simulink model "playback_data"  (R2015a)
settings: Solver=FixedStepDiscrete  SolverMode=SingleTasking  StartTime=76  StopTime=110  FixedStep=sample_time  RelTol=1e-3
undefined symbols (not defined in the file): A1_notch_f1, A2_notch_f1, A_kalman_swing_load, A_kalman_transverse, A_kalman_vertical, A_lpf_accelerometer, A_lpf_dtau, A_lpf_fourbar_angles, A_lpf_imu, A_lpf_lateral_angle, B1_lpf_accelerometer, B1_lpf_dtau, B1_lpf_fourbar_angles, B1_lpf_imu, B1_lpf_lateral_angle, B1_notch_f1, B2_lpf_accelerometer, B2_lpf_dtau, B2_lpf_fourbar_angles, B2_lpf_imu, B2_lpf_lateral_angle, B2_notch_f1, B_dx_versus_x0, B_kalman_swing_load, B_kalman_transverse, B_kalman_vertical, backwards_K_sag_of_t, backwards_P_sag_of_t, C_kalman_swing_load, C_kalman_transverse, C_kalman_vertical, com_leg_motor, com_torso, contact_threshold, control_start_time, d_ankle_to_foot, d_vertical_com, desired_com_forward_velocity, desired_com_lateral_velocity, desired_initial_leg_roll_left, desired_initial_leg_roll_right, desired_stance_beta2, desired_standing_torso_pitch, desired_standing_torso_roll, desired_standing_z, desired_torso_pitch, desired_torso_roll, Discrete, enable_bouncing, fcut_contact, fdesignblkfcn, forward_dx_of_dxstar, forward_x_of_dxstar, g, gcbh, HIP_MTR_MAX_CONT_TORQUE, HIP_MTR_MAX_TORQUE, i_leg_motor, i_robot, i_torso ... (+78)
libraries: simulink x65, dsparch4 x18, ctrlSharedLib x14, dspfdesign x4
(part 7 of 13)

== system playback_data/Control/Actuator Control with Torque SEA commands/SEA Controller (Velocity)/Lowpass Filter (Stance) ==
  In : Inport
  Generated Filter Block : DiscreteFir  Tag=BlockMethodSubSystem  Coefficients=[-0.049792265798371309 -0.00478204397482343 -0.0023545966524627579 0.0019617877955006649 0.0081617445920188422 0.01606136498204886 0.025426522925330174 0.035808512742994333 0.046780148761454213 0.057713212050140641 0.068077289761393753 0.077169075575072327 0.084565882051693325 0.089692876147162801 0.092473878579640248 0.092473878579640248 0.089692876147162801 0.084565882051693325 0.077169075575072327 0.068077289761393753 0.057713212050140641 0.046780148761454213 0.035808512742994333 0.025426522925330174 0.01606136498204886 0.0081617445920188422 0.0019617877955006649 -0.0023545966524627579 -0.00478204397482343 -0.049792265798371309]
  Out : Outport
  wires:
  In/1 -> Generated Filter Block/1
  Generated Filter Block/1 -> Out/1

== system playback_data/Control/Actuator Control with Torque SEA commands/SEA Controller (Velocity)/Lowpass Filter (Swing) ==
  In : Inport
  Generated Filter Block : dsparch4/Biquad Filter  Tag=BlockMethodSubSystem  IIRFiltStruct=Direct form II  CoeffSource=Specify via dialog  BiQuadCoeffs=[1.0218648663828083 -2 1.0218648663828083 1 -1.9114378222117407 0.91557643487411833]  a0Flag=Warning  IC=0  ICnum=0  ICden=0  denAccumFracLength=30  denProdOutputFracLength=30  secondMemoryFracLength=15  roundingMode=Floor  overflowMode=off  ScaleValues=[0.0041174265739107223;22.985401576126357]  optimizeScaleValues=off  ScaleValueMode=Specify via input port (g)  scaleValueFracLength=14  FilterSource=Specify via dialog  FilterObject=Hm_biquad
  Out : Outport
  wires:
  Generated Filter Block/1 -> Out/1
  In/1 -> Generated Filter Block/1

== system playback_data/Control/Actuator Control with Torque SEA commands/SEA Controller (Velocity)/Stance or Swing ==
  True/False x4 : Inport
  Signal True x4 : Inport  Port=2
  Signal False x4 : Inport  Port=3
  Demux : Demux
  Demux1 : Demux
  Demux2 : Demux
  Mux : Mux
  Switch{,1..3} (4 alike) : Switch  Criteria=u2 ~= 0
  Selected x4 : Outport
  wires:
  Mux/1 -> Selected x4/1
  True/False x4/1 -> Demux1/1
  Signal True x4/1 -> Demux/1
  Signal False x4/1 -> Demux2/1
  Demux/1 -> Switch/1
  Demux/2 -> Switch1/1
  Demux/3 -> Switch2/1
  Demux/4 -> Switch3/1
  Demux2/1 -> Switch/3
  Demux2/2 -> Switch1/3
  Demux2/3 -> Switch2/3
  Demux2/4 -> Switch3/3
  Demux1/1 -> Switch/2
  Demux1/2 -> Switch1/2
  Demux1/3 -> Switch2/2
  Demux1/4 -> Switch3/2
  Switch/1 -> Mux/1
  Switch1/1 -> Mux/2
  Switch2/1 -> Mux/3
  Switch3/1 -> Mux/4

== system playback_data/Control/Actuator Control with Torque SEA commands/SEA Controller (Velocity)/Stance or Swing1 ==
  True/False x4 : Inport
  Signal True x4 : Inport  Port=2
  Signal False x4 : Inport  Port=3
  Demux : Demux
  Demux1 : Demux
  Demux2 : Demux
  Mux : Mux
  Switch{,1..3} (4 alike) : Switch  Criteria=u2 ~= 0
  Selected x4 : Outport
  wires:
  Switch3/1 -> Mux/4
  Switch2/1 -> Mux/3
  Switch1/1 -> Mux/2
  Switch/1 -> Mux/1
  Demux1/4 -> Switch3/2
  Demux1/3 -> Switch2/2
  Demux1/2 -> Switch1/2
  Demux1/1 -> Switch/2
  Demux2/4 -> Switch3/3
  Demux2/3 -> Switch2/3
  Demux2/2 -> Switch1/3
  Demux2/1 -> Switch/3
  Demux/4 -> Switch3/1
  Demux/3 -> Switch2/1
  Demux/2 -> Switch1/1
  Demux/1 -> Switch/1
  Signal False x4/1 -> Demux2/1
  Signal True x4/1 -> Demux/1
  True/False x4/1 -> Demux1/1
  Mux/1 -> Selected x4/1

== system playback_data/Control/Actuator Control with Torque SEA commands/SEA Controller (Velocity)/Stance or Swing2 ==
  True/False x4 : Inport
  Signal True x4 : Inport  Port=2
  Signal False x4 : Inport  Port=3
  Demux : Demux
  Demux1 : Demux
  Demux2 : Demux
  Mux : Mux
  Switch{,1..3} (4 alike) : Switch  Criteria=u2 ~= 0
  Selected x4 : Outport
  wires:
  Mux/1 -> Selected x4/1
  True/False x4/1 -> Demux1/1
  Signal True x4/1 -> Demux/1
  Signal False x4/1 -> Demux2/1
  Demux/1 -> Switch/1
  Demux/2 -> Switch1/1
  Demux/3 -> Switch2/1
  Demux/4 -> Switch3/1
  Demux2/1 -> Switch/3
  Demux2/2 -> Switch1/3
  Demux2/3 -> Switch2/3
  Demux2/4 -> Switch3/3
  Demux1/1 -> Switch/2
  Demux1/2 -> Switch1/2
  Demux1/3 -> Switch2/2
  Demux1/4 -> Switch3/2
  Switch/1 -> Mux/1
  Switch1/1 -> Mux/2
  Switch2/1 -> Mux/3
  Switch3/1 -> Mux/4

== system playback_data/Control/Actuator Control with Torque SEA commands/Timers/Time on Contact ==
  in : Inport
  Trigger : TriggerPort  ShowOutputPort=on  PortDimensions=1
  Subsystem : Subsystem
  out : Outport
  wires:
  in/1 -> Subsystem/1(in)
  Subsystem/1(out) -> out/1
  Trigger/1 -> Subsystem/Enable

== system playback_data/Control/Actuator Control with Torque SEA commands/Timers/Time on Contact1 ==
  in : Inport
  Trigger : TriggerPort  ShowOutputPort=on  PortDimensions=1
  Subsystem : Subsystem
  out : Outport
  wires:
  Trigger/1 -> Subsystem/Enable
  Subsystem/1(out) -> out/1
  in/1 -> Subsystem/1(in)

== system playback_data/Control/Actuator Control with Torque SEA commands/Timers/Time on Contact2 ==
  in : Inport
  Trigger : TriggerPort  ShowOutputPort=on  PortDimensions=1
  Subsystem : Subsystem
  out : Outport
  wires:
  Trigger/1 -> Subsystem/Enable
  Subsystem/1(out) -> out/1
  in/1 -> Subsystem/1(in)

== system playback_data/Control/Actuator Control with Torque SEA commands/Timers/Time on Contact3 ==
  in : Inport
  Trigger : TriggerPort  ShowOutputPort=on  PortDimensions=1
  Subsystem : Subsystem
  out : Outport
  wires:
  in/1 -> Subsystem/1(in)
  Subsystem/1(out) -> out/1
  Trigger/1 -> Subsystem/Enable

== system playback_data/Control/Behavior Control/Force Estimation/Leg Force Measurements ==
  q : Inport
  Leg Width Right/Left [m m] : Inport  Port=2
  Leg Length Right/Left [m m] : Inport  Port=3
  Demux : Demux  Outputs=2
  Demux1 : Demux  Outputs=2
  Demux2 : Demux
  Divide{1..4} (4 alike) : Product  Inputs=*/
  Gain : Gain  Commented=on  Gain=k_sea_low
  Mux : Mux
  Nonlinear Spring Force : MATLAB Function  TreatAsAtomicUnit=on
  Sum{1..3,6} (4 alike) : Sum  Inputs=-+|
  Sum4 : Sum  Inputs=-|+
  Sum5 : Sum  Inputs=-|+
  Sum7 : Sum  Inputs=+|+
  Sum8 : Sum  Inputs=+|+
  backGearL : Selector  InputPortWidth=13  Indices=[6]
  backGearR : Selector  InputPortWidth=13  Indices=[2]
  backJointL : Selector  InputPortWidth=13  Indices=[5]
  backJointR : Selector  InputPortWidth=13  Indices=[1]
  frontGearL : Selector  InputPortWidth=13  Indices=[8]
  frontGearR : Selector  InputPortWidth=13  Indices=[4]
  frontJointL : Selector  InputPortWidth=13  Indices=[7]
  frontJointR : Selector  InputPortWidth=13  Indices=[3]
  Right Leg Torque [Nm] : Outport
  Left Leg Torque [Nm] : Outport  Port=2
  Right Leg Axial Force [N] : Outport  Port=3
  Left Leg Axial Force [N] : Outport  Port=4
  Right Leg Orthogonal Force [N] : Outport  Port=5
  Left Leg Orthogonal Force [N] : Outport  Port=6
  wires:
  Sum3/1 -> Mux/4
  Sum2/1 -> Mux/3
  backJointL/1 -> Sum2/1
  frontGearL/1 -> Sum3/2
  frontJointL/1 -> Sum3/1
  backGearL/1 -> Sum2/2
  Sum6/1 -> Mux/1
  Sum1/1 -> Mux/2
  backJointR/1 -> Sum6/1
  frontGearR/1 -> Sum1/2
  frontJointR/1 -> Sum1/1
  backGearR/1 -> Sum6/2
  q/1 -> backGearR/1, backJointL/1, frontJointL/1, frontGearL/1, backGearL/1, frontGearR/1, frontJointR/1, backJointR/1
  Demux2/1 -> Sum4/1, Sum7/1
  Demux2/2 -> Sum7/2, Sum4/2
  Demux2/4 -> Sum5/2, Sum8/2
  Sum4/1 -> Divide1/1
  Sum5/1 -> Divide2/1
  Leg Width Right/Left [m m]/1 -> Demux/1
  Demux/1 -> Divide1/2
  Demux/2 -> Divide2/2
  Divide1/1 -> Right Leg Axial Force [N]/1
  Divide2/1 -> Left Leg Axial Force [N]/1
  Demux2/3 -> Sum8/1, Sum5/1
  Sum7/1 -> Divide3/1, Right Leg Torque [Nm]/1
  Sum8/1 -> Divide4/1, Left Leg Torque [Nm]/1
  Demux1/1 -> Divide3/2
  Demux1/2 -> Divide4/2
  Leg Length Right/Left [m m]/1 -> Demux1/1
  Divide3/1 -> Right Leg Orthogonal Force [N]/1
  Divide4/1 -> Left Leg Orthogonal Force [N]/1
  Mux/1 -> Nonlinear Spring Force/1(deflections)
  Nonlinear Spring Force/1(tau_sea) -> Demux2/1

== system playback_data/Control/Behavior Control/Force Estimation/Leg Plane GRF ==
  Axial Force [N] : Inport
  Orthogonal Force [N] : Inport  Port=2
  Torso Pitch [rad] : Inport  Port=3
  Leg Angle [rad] : Inport  Port=4
  Gain : Gain  Gain=-1
  Product : Product
  Product1 : Product
  Sum : Sum  Inputs=++|
  Sum1 : Sum  Inputs=+|+
  Trigonometric Function : Trigonometry  Operator=cos
  Trigonometric Function1 : Trigonometry
  Vertical Force [N] : Outport
  wires:
  Product1/1 -> Sum1/2
  Sum1/1 -> Vertical Force [N]/1
  Trigonometric Function1/1 -> Product1/2
  Orthogonal Force [N]/1 -> Product1/1
  Axial Force [N]/1 -> Product/1
  Leg Angle [rad]/1 -> Sum/2
  Torso Pitch [rad]/1 -> Sum/1
  Trigonometric Function/1 -> Product/2
  Product/1 -> Gain/1
  Sum/1 -> Trigonometric Function/1, Trigonometric Function1/1
  Gain/1 -> Sum1/1

== system playback_data/Control/Behavior Control/Primary and Lateral Behavior/Circular Buffer ==
  Flight [1/0] : Inport
  Exiting Stance [1/0] : Inport  Port=2
  Hopping [1/0] : Inport  Port=3
  dX [m/s] : Inport  Port=4
  dY [m/s] : Inport  Port=5
  X Foot Correction [m] : Inport  Port=6
  Y Foot Correction [m] : Inport  Port=7
  target dX [m/s] : Inport  Port=8
  target dY [m/s] : Inport  Port=9
  Buffer : MATLAB Function  TreatAsAtomicUnit=on  SystemSampleTime=sample_time
  Buffer1 : MATLAB Function  TreatAsAtomicUnit=on  SystemSampleTime=sample_time
  Buffer2 : MATLAB Function  TreatAsAtomicUnit=on  SystemSampleTime=sample_time
  Buffer3 : MATLAB Function  TreatAsAtomicUnit=on  SystemSampleTime=sample_time
  Buffer4 : MATLAB Function  TreatAsAtomicUnit=on  SystemSampleTime=sample_time
  Buffer5 : MATLAB Function  TreatAsAtomicUnit=on  SystemSampleTime=sample_time
  Buffer6 : MATLAB Function  TreatAsAtomicUnit=on  SystemSampleTime=sample_time
  Buffer7 : MATLAB Function  TreatAsAtomicUnit=on  SystemSampleTime=sample_time
  Demux : Demux  Outputs=6
  Detect Decrease : simulink/Logic and Bit Operations/Detect Decrease  vinit=0.0  InputProcessing=Inherited  OutDataTypeStr=boolean
  Enabled on Touchdown : Subsystem  TreatAsAtomicUnit=on
  Logical Operator : Logic  AllPortsSameDT=off  OutDataTypeStr=boolean
  Mux : Mux  Inputs=6
  buffer size5 : Constant  Value=recorded_steps
  "dX Touchdown History " : Outport
  X Foot Correction History : Outport  Port=2
  dX Takeoff History : Outport  Port=3
  "dY Touchdown History " : Outport  Port=4
  Y Foot Correction History : Outport  Port=5
  dY Takeoff History : Outport  Port=6
  target dX History : Outport  Port=7
  target dY History : Outport  Port=8
  wires:
  Enabled on Touchdown/1(Out) -> Demux/1
  Mux/1 -> Enabled on Touchdown/1(In)
  Logical Operator/1 -> Detect Decrease/1
  Flight [1/0]/1 -> Logical Operator/2
  dX [m/s]/1 -> Mux/1, Buffer2/1(data)
  dY [m/s]/1 -> Mux/2, Buffer5/1(data)
  Hopping [1/0]/1 -> Logical Operator/1
  Exiting Stance [1/0]/1 -> Buffer5/2(trigger), Buffer2/2(trigger), Buffer3/2(trigger), Buffer1/2(trigger), Buffer4/2(trigger), Buffer6/2(trigger), Buffer7/2(trigger), Buffer/2(trigger)
  target dY [m/s]/1 -> Mux/6
  Demux/5 -> Buffer6/1(data)
  Demux/6 -> Buffer7/1(data)
  buffer size5/1 -> Buffer5/3(buffer_size), Buffer3/3(buffer_size), Buffer1/3(buffer_size), Buffer4/3(buffer_size), Buffer6/3(buffer_size), Buffer7/3(buffer_size), Buffer/3(buffer_size), Buffer2/3(buffer_size)
  Buffer7/1(buffer) -> target dY History/1
  Buffer6/1(buffer) -> target dX History/1
  target dX [m/s]/1 -> Mux/5
  Demux/4 -> Buffer4/1(data)
  Y Foot Correction [m]/1 -> Mux/4
  Buffer5/1(buffer) -> dY Takeoff History/1
  Demux/2 -> Buffer3/1(data)
  Buffer4/1(buffer) -> Y Foot Correction History/1
  Buffer3/1(buffer) -> "dY Touchdown History "/1
  X Foot Correction [m]/1 -> Mux/3
  Demux/3 -> Buffer1/1(data)
  Demux/1 -> Buffer/1(data)
  Buffer2/1(buffer) -> dX Takeoff History/1
  Buffer1/1(buffer) -> X Foot Correction History/1
  Detect Decrease/1 -> Enabled on Touchdown/Enable
  Buffer/1(buffer) -> "dX Touchdown History "/1

== system playback_data/Control/Behavior Control/Primary and Lateral Behavior/Closed Loop Compensation ==
  dX Touchdown History : Inport
  X Foot Correction History : Inport  Port=2
  dX Takeoff History : Inport  Port=3
  dY Touchdown History : Inport  Port=4
  Y Foot Correction History : Inport  Port=5
  dY Takeoff History : Inport  Port=6
  target dX History : Inport  Port=7
  target dY History : Inport  Port=8
  dX [m/s] : Inport  Port=9
  dY [m/s] : Inport  Port=10
  target dX [m/s] : Inport  Port=11
  "target dY [m/s] " : Inport  Port=12
  A_x : Gain
  A_x_no_bias : Gain
  A_y : Gain
  A_y_no_bias : Gain
  CLOSED LOOP COMPENSATION X FOR VAIRABLE SPEED : MATLAB Function  TreatAsAtomicUnit=on
  CLOSED LOOP COMPENSATION Y FOR VAIRABLE SPEED : MATLAB Function  TreatAsAtomicUnit=on
  Constant4 : Constant  Value=B_dx_versus_x0
  ESTIMATE CLOSED LOOP ERROR X FOR VARIABLE SPEED : MATLAB Function  TreatAsAtomicUnit=on
  ESTIMATE CLOSED LOOP ERROR Y FOR VARIABLE SPEED : MATLAB Function  TreatAsAtomicUnit=on
  How much dx depends on x0 : Constant  Value=B_dx_versus_x0
  RealVsFakeWeight : Constant  Value=2
  RealVsFakeWeight1 : Constant  Value=2
  Sum : Sum  Inputs=|+-
  Sum1 : Sum  Inputs=|+-
  Terminator{2..12,14} (12 alike) : Terminator
  XY Foot Correction : Scope  NumInputPorts=2
      settings: YMin=-1~-0.8  YMax=1~1.4  SaveName=ScopeData39  SampleInput=on
  c_x : Gain
  c_x_no_bias : Gain
  c_y : Gain
  c_y_no_bias : Gain
  epsilon_x : Gain
  epsilon_x_no_bias : Gain
  epsilon_y : Gain
  epsilon_y_no_bias : Gain
  X Foot Correction [m] : Outport
  Y Foot Correction [m] : Outport  Port=2
  wires:
  RealVsFakeWeight1/1 -> ESTIMATE CLOSED LOOP ERROR Y FOR VARIABLE SPEED/5(W_real)
  Constant4/1 -> CLOSED LOOP COMPENSATION Y FOR VAIRABLE SPEED/6(B_cl)
  "target dY [m/s] "/1 -> Sum1/2, CLOSED LOOP COMPENSATION Y FOR VAIRABLE SPEED/5(dx_star)
  target dY History/1 -> ESTIMATE CLOSED LOOP ERROR Y FOR VARIABLE SPEED/4(dx_star_hist)
  Y Foot Correction History/1 -> ESTIMATE CLOSED LOOP ERROR Y FOR VARIABLE SPEED/2(delta_ux_hist)
  dY Takeoff History/1 -> ESTIMATE CLOSED LOOP ERROR Y FOR VARIABLE SPEED/3(dx_lift_hist)
  dY [m/s]/1 -> Sum1/1
  RealVsFakeWeight/1 -> ESTIMATE CLOSED LOOP ERROR X FOR VARIABLE SPEED/5(W_real)
  How much dx depends on x0/1 -> CLOSED LOOP COMPENSATION X FOR VAIRABLE SPEED/6(B_cl)
  Sum/1 -> CLOSED LOOP COMPENSATION X FOR VAIRABLE SPEED/4(delta_s_i)
  target dX [m/s]/1 -> Sum/2, CLOSED LOOP COMPENSATION X FOR VAIRABLE SPEED/5(dx_star)
  target dX History/1 -> ESTIMATE CLOSED LOOP ERROR X FOR VARIABLE SPEED/4(dx_star_hist)
  X Foot Correction History/1 -> ESTIMATE CLOSED LOOP ERROR X FOR VARIABLE SPEED/2(delta_ux_hist)
  dX Takeoff History/1 -> ESTIMATE CLOSED LOOP ERROR X FOR VARIABLE SPEED/3(dx_lift_hist)
  dX Touchdown History/1 -> ESTIMATE CLOSED LOOP ERROR X FOR VARIABLE SPEED/1(dx_land_hist)
  dX [m/s]/1 -> Sum/1
  dY Touchdown History/1 -> ESTIMATE CLOSED LOOP ERROR Y FOR VARIABLE SPEED/1(dx_land_hist)
  Sum1/1 -> CLOSED LOOP COMPENSATION Y FOR VAIRABLE SPEED/4(delta_s_i)
  CLOSED LOOP COMPENSATION X FOR VAIRABLE SPEED/1(delta_ux) -> XY Foot Correction/1, X Foot Correction [m]/1
  CLOSED LOOP COMPENSATION Y FOR VAIRABLE SPEED/1(delta_ux) -> XY Foot Correction/2, Y Foot Correction [m]/1
  ESTIMATE CLOSED LOOP ERROR X FOR VARIABLE SPEED/6(c_nb) -> c_x_no_bias/1
  ESTIMATE CLOSED LOOP ERROR X FOR VARIABLE SPEED/5(epsilon_0_nb) -> epsilon_x_no_bias/1
  ESTIMATE CLOSED LOOP ERROR X FOR VARIABLE SPEED/4(A_cl_nb) -> A_x_no_bias/1
  A_x_no_bias/1 -> Terminator5/1
  epsilon_x_no_bias/1 -> Terminator6/1
  c_x_no_bias/1 -> Terminator7/1
  A_y_no_bias/1 -> Terminator2/1
  epsilon_y_no_bias/1 -> Terminator3/1
  c_y_no_bias/1 -> Terminator4/1
  ESTIMATE CLOSED LOOP ERROR Y FOR VARIABLE SPEED/4(A_cl_nb) -> A_y_no_bias/1
  ESTIMATE CLOSED LOOP ERROR Y FOR VARIABLE SPEED/5(epsilon_0_nb) -> epsilon_y_no_bias/1
  ESTIMATE CLOSED LOOP ERROR Y FOR VARIABLE SPEED/6(c_nb) -> c_y_no_bias/1
  ESTIMATE CLOSED LOOP ERROR X FOR VARIABLE SPEED/3(c) -> c_x/1, CLOSED LOOP COMPENSATION X FOR VAIRABLE SPEED/3(c)
  ESTIMATE CLOSED LOOP ERROR X FOR VARIABLE SPEED/2(epsilon_0) -> epsilon_x/1, CLOSED LOOP COMPENSATION X FOR VAIRABLE SPEED/2(epsilon)
  ESTIMATE CLOSED LOOP ERROR X FOR VARIABLE SPEED/1(A_cl) -> A_x/1, CLOSED LOOP COMPENSATION X FOR VAIRABLE SPEED/1(A_cl)
  A_x/1 -> Terminator8/1
  epsilon_x/1 -> Terminator9/1
  c_x/1 -> Terminator10/1
  ESTIMATE CLOSED LOOP ERROR Y FOR VARIABLE SPEED/3(c) -> c_y/1, CLOSED LOOP COMPENSATION Y FOR VAIRABLE SPEED/3(c)
  ESTIMATE CLOSED LOOP ERROR Y FOR VARIABLE SPEED/2(epsilon_0) -> epsilon_y/1, CLOSED LOOP COMPENSATION Y FOR VAIRABLE SPEED/2(epsilon)
  ESTIMATE CLOSED LOOP ERROR Y FOR VARIABLE SPEED/1(A_cl) -> A_y/1, CLOSED LOOP COMPENSATION Y FOR VAIRABLE SPEED/1(A_cl)
  A_y/1 -> Terminator12/1
  epsilon_y/1 -> Terminator14/1
  c_y/1 -> Terminator11/1

== system playback_data/Control/Behavior Control/Primary and Lateral Behavior/Enabled on Takeoff ==
  In : Inport
  Enable : EnablePort
  Out : Outport
  wires:
  In/1 -> Out/1

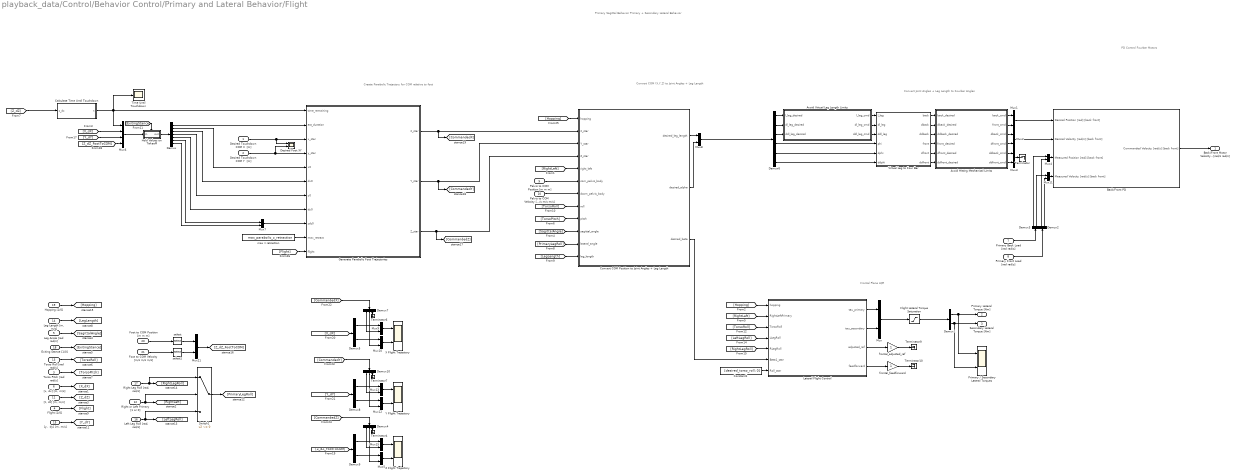
== system playback_data/Control/Behavior Control/Primary and Lateral Behavior/Flight ==
  note: Primary Sagittal Behavior
      | Primary + Secondary Lateral Behavior
  note: Create Parabolic
      | Trajectory for COM relative to foot
  note: Convert COM (X,Y,Z) to
      | Joint Angles + Leg Length
  note: Convert Joint Angles + Leg Length
      | to Fourbar Angles
  note: PD Control Fourbar Motors
  note: Frontal Plane LQR
  Desired Touchdown COM X  [m] : Inport
  Desired Touchdown COM Y  [m] : Inport  Port=2
  Torso Pitch [rad rad/s] : Inport  Port=3
  Flight [1/0] : Inport  Port=4
  Leg Angle [rad rad/s] : Inport  Port=5
  "[x, dx] [m, m/s]" : Inport  Port=6
  Primary Back Load [rad rad/s] : Inport  Port=7
  Primary Front Load [rad rad/s] : Inport  Port=8
  Pelvis to COM Position [m m m] : Inport  Port=9
  Pelvis to COM Velocity [m/s m/s m/s] : Inport  Port=10
  "[z, dz] [m, m/s]" : Inport  Port=11
  Right or Left Primary [1 or 0] : Inport  Port=12
  Torso Roll [rad rad/s] : Inport  Port=13
  "Leg Length [m, m/s]" : Inport  Port=14
  "[y,  dy] [m, m/s]" : Inport  Port=15
  "Left Leg Roll [rad, rad/s]" : Inport  Port=16
  "Right Leg Roll [rad, rad/s]" : Inport  Port=17
  Exiting Stance [1/0] : Inport  Port=18
  Hopping [1/0] : Inport  Port=19
  Foot to COM Position [m m m] : Inport  Port=20
  Foot to COM Velocity [m/s m/s m/s] : Inport  Port=21
  Avoid Hitting Mechanical Limits : MATLAB Function  TreatAsAtomicUnit=on
  Avoid Virtual Leg Length Limits : MATLAB Function  TreatAsAtomicUnit=on
  Back/Front PD : Subsystem
  Calculate Time Until Touchdown : MATLAB Function  TreatAsAtomicUnit=on
  Constant1 : Constant  Value=[desired_torso_roll; 0]
  "Convert COM Position to Joint Angles + Leg Length " : MATLAB Function  TreatAsAtomicUnit=on
  Demux : Demux  Outputs=7
  Demux{1..3,5,8..9} (6 alike) : Demux  Outputs=2
  Demux10 : Demux  Outputs=3
  Demux4 : Demux  Outputs=3
  Demux6 : Demux  Outputs=6
  Demux7 : Demux  Outputs=3
  Desired Foot XY : Scope  NumInputPorts=2
      settings: YMin=-1~-0.8  YMax=1~1.4  SaveName=ScopeData38  SampleInput=on
  Flight Lateral Torque Saturation : Saturate  UpperLimit=HIP_MTR_MAX_CONT_TORQUE  LowerLimit=-HIP_MTR_MAX_CONT_TORQUE
      settings: AttributesFormatString=Top: %<UpperLimit>\nBottom: %<LowerLimit>
  Generate Parabolic Foot Trajectories : MATLAB Function  TreatAsAtomicUnit=on
  Hold Values on Takeoff : Subsystem
  Lateral Flight Control : MATLAB Function  TreatAsAtomicUnit=on
  Mux{,1..5,7..13,15,21} (15 alike) : Mux  Inputs=2
  Mux6 : Mux
  Primary / Secondary Lateral Torques : Scope  NumInputPorts=2
      settings: YMin=-1~-0.8  YMax=1~1.4  SaveName=ScopeData32  SampleInput=on
  Switch1 : Switch  Criteria=u2 ~= 0
  Terminator{,4,6..7,9..10} (6 alike) : Terminator
  Time Until Touchdown : Scope
      settings: YMin=-1  YMax=1  SaveName=ScopeData37  SampleInput=on
  Virtual Leg to Four Bar : MATLAB Function  TreatAsAtomicUnit=on
  X Flight Trajectory : Scope  NumInputPorts=2
      settings: YMin=-1~-0.8  YMax=1~1.4  SaveName=ScopeData3  SampleInput=on
  Y Flight Trajectory : Scope  NumInputPorts=2
      settings: YMin=-1~-0.8  YMax=1~1.4  SaveName=ScopeData4  SampleInput=on
  Z Flight Trajectory : Scope  NumInputPorts=2
      settings: YMin=-1~-0.8  YMax=1~1.4  SaveName=ScopeData7  SampleInput=on
  frontal_adjusted_ref : Gain
  frontal_feedforward : Gain
  max z retraction : Constant  Value=max_parabolic_z_retraction
  select : Selector  InputPortWidth=3  Indices=[3]
  select1 : Selector  InputPortWidth=3  Indices=[3]
  Back/Front Motor Velocity [rad/s rad/s] : Outport
  Primary Lateral Torque [Nm] : Outport  Port=2
  Secondary Lateral Torque [Nm] : Outport  Port=3
  wires:
  Virtual Leg to Four Bar/1(back) -> Avoid Hitting Mechanical Limits/1(back_desired)
  Virtual Leg to Four Bar/2(dback) -> Avoid Hitting Mechanical Limits/2(dback_desired)
  Virtual Leg to Four Bar/3(ddback) -> Avoid Hitting Mechanical Limits/3(ddback_desired)
  Virtual Leg to Four Bar/4(front) -> Avoid Hitting Mechanical Limits/4(front_desired)
  Virtual Leg to Four Bar/5(dfront) -> Avoid Hitting Mechanical Limits/5(dfront_desired)
  Virtual Leg to Four Bar/6(ddfront) -> Avoid Hitting Mechanical Limits/6(ddfront_desired)
  Mux11/1 -> Back/Front PD/4(Measured Velocity [rad/s] [back front])
  Demux2/2 -> Mux11/2
  Mux4/1 -> Back/Front PD/3(Measured Position [rad] [back front])
  Mux1/1 -> Back/Front PD/1(Desired Position [rad] [back front])
  Demux3/2 -> Mux11/1
  Demux3/1 -> Mux4/1
  Avoid Hitting Mechanical Limits/2(front_cmd) -> Mux1/2
  Avoid Hitting Mechanical Limits/1(back_cmd) -> Mux1/1
  Demux2/1 -> Mux4/2
  Avoid Hitting Mechanical Limits/3(dback_cmd) -> Mux2/1
  Avoid Hitting Mechanical Limits/4(dfront_cmd) -> Mux2/2
  Avoid Hitting Mechanical Limits/5(ddback_cmd) -> Mux3/1
  Avoid Hitting Mechanical Limits/6(ddfront_cmd) -> Mux3/2
  Mux2/1 -> Back/Front PD/2(Desired Velocity [rad/s] [back front])
  Back/Front PD/1(Commanded Velocity [rad/s] [back front]) -> Back/Front Motor Velocity [rad/s rad/s]/1
  Primary Back Load [rad rad/s]/1 -> Demux3/1
  Primary Front Load [rad rad/s]/1 -> Demux2/1
  Demux/1 -> Generate Parabolic Foot Trajectories/2(est_duration)
  Mux7/1 -> Generate Parabolic Foot Trajectories/9(zdz0)
  max z retraction/1 -> Generate Parabolic Foot Trajectories/10(max_retract)
  Mux6/1 -> Hold Values on Takeoff/1(in)
  Hold Values on Takeoff/1(out) -> Demux/1
  [X_dX] -> Mux6/2
  Generate Parabolic Foot Trajectories/1(X_star) -> [CommandedX], "Convert COM Position to Joint Angles + Leg Length "/2(X_star)
  Generate Parabolic Foot Trajectories/2(Y_star) -> "Convert COM Position to Joint Angles + Leg Length "/3(Y_star), [CommandedY]
  [RightLeft] -> "Convert COM Position to Joint Angles + Leg Length "/5(right_left)
  "Convert COM Position to Joint Angles + Leg Length "/2(desired_alpha) -> Mux8/2
  "Convert COM Position to Joint Angles + Leg Length "/1(desired_leg_length) -> Mux8/1
  Demux6/6 -> Virtual Leg to Four Bar/6(ddphi)
  Demux6/5 -> Virtual Leg to Four Bar/5(dphi)
  Demux6/4 -> Virtual Leg to Four Bar/4(phi)
  Mux8/1 -> Demux6/1
  Leg Angle [rad rad/s]/1 -> [SagittalAngle]
  [SagittalAngle] -> "Convert COM Position to Joint Angles + Leg Length "/10(sagittal_angle)
  Torso Pitch [rad rad/s]/1 -> [TorsoPitch]
  [TorsoPitch] -> "Convert COM Position to Joint Angles + Leg Length "/9(pitch)
  [PrimaryLegRoll] -> "Convert COM Position to Joint Angles + Leg Length "/11(lateral_angle)
  [LegLength] -> "Convert COM Position to Joint Angles + Leg Length "/12(leg_length)
  [TorsoRoll] -> "Convert COM Position to Joint Angles + Leg Length "/8(roll)
  Pelvis to COM Position [m m m]/1 -> "Convert COM Position to Joint Angles + Leg Length "/6(com_pelvis_body)
  Pelvis to COM Velocity [m/s m/s m/s]/1 -> "Convert COM Position to Joint Angles + Leg Length "/7(dcom_pelvis_body)
  Flight [1/0]/1 -> [Flight]
  [ExitingStance] -> Hold Values on Takeoff/Trigger
  "[x, dx] [m, m/s]"/1 -> [X_dX]
  Torso Roll [rad rad/s]/1 -> [TorsoRoll]
  "Leg Length [m, m/s]"/1 -> [LegLength]
  "[z, dz] [m, m/s]"/1 -> [Z_dZ]
  Desired Touchdown COM X  [m]/1 -> Desired Foot XY/1, Generate Parabolic Foot Trajectories/3(x_star)
  "[y,  dy] [m, m/s]"/1 -> [Y_dY]
  [Y_dY] -> Mux6/3
  [Z_dZ] -> Calculate Time Until Touchdown/1(z_dz)
  Calculate Time Until Touchdown/1(t) -> Mux6/1, Time Until Touchdown/1, Generate Parabolic Foot Trajectories/1(time_remaining)
  Avoid Virtual Leg Length Limits/1(l_leg_cmd) -> Virtual Leg to Four Bar/1(l_leg)
  Avoid Virtual Leg Length Limits/2(dl_leg_cmd) -> Virtual Leg to Four Bar/2(dl_leg)
  Avoid Virtual Leg Length Limits/3(ddl_leg_cmd) -> Virtual Leg to Four Bar/3(ddl_leg)
  Demux6/1 -> Avoid Virtual Leg Length Limits/1(l_leg_desired)
  Demux6/2 -> Avoid Virtual Leg Length Limits/2(dl_leg_desired)
  Demux6/3 -> Avoid Virtual Leg Length Limits/3(ddl_leg_desired)
  Desired Touchdown COM Y  [m]/1 -> Desired Foot XY/2, Generate Parabolic Foot Trajectories/4(y_star)
  [RightLeft] -> Lateral Flight Control/2(RightLeftPrimary)
  [TorsoRoll] -> Lateral Flight Control/3(TorsoRoll)
  Constant1/1 -> Lateral Flight Control/7(Roll_star)
  Lateral Flight Control/3(adjusted_ref) -> frontal_adjusted_ref/1
  Lateral Flight Control/4(feedforward) -> frontal_feedforward/1
  Lateral Flight Control/2(tau_secondary) -> Mux/2
  Lateral Flight Control/1(tau_primary) -> Mux/1
  "Left Leg Roll [rad, rad/s]"/1 -> Switch1/3, [LeftLegRoll]
  [LeftLegRoll] -> Lateral Flight Control/4(LLegRoll)
  [RightLegRoll] -> Lateral Flight Control/5(RLegRoll)
  "Right Leg Roll [rad, rad/s]"/1 -> Switch1/1, [RightLegRoll]
  Right or Left Primary [1 or 0]/1 -> Switch1/2, [RightLeft]
  Switch1/1 -> [PrimaryLegRoll]
  Exiting Stance [1/0]/1 -> [ExitingStance]
  Demux1/1 -> Primary / Secondary Lateral Torques/1, Primary Lateral Torque [Nm]/1
  Demux1/2 -> Primary / Secondary Lateral Torques/2, Secondary Lateral Torque [Nm]/1
  "Convert COM Position to Joint Angles + Leg Length "/3(desired_beta) -> Lateral Flight Control/6(Beta1_star)
  Flight Lateral Torque Saturation/1 -> Demux1/1
  frontal_feedforward/1 -> Terminator10/1
  frontal_adjusted_ref/1 -> Terminator9/1
  [Hopping] -> "Convert COM Position to Joint Angles + Leg Length "/1(hopping)
  Mux/1 -> Flight Lateral Torque Saturation/1
  [Hopping] -> Lateral Flight Control/1(hopping)
  Hopping [1/0]/1 -> [Hopping]
  [Flight] -> Generate Parabolic Foot Trajectories/11(flight)
  Demux/2 -> Generate Parabolic Foot Trajectories/5(x0)
  Demux/3 -> Generate Parabolic Foot Trajectories/6(dx0)
  Demux/4 -> Generate Parabolic Foot Trajectories/7(y0)
  Demux/5 -> Generate Parabolic Foot Trajectories/8(dy0)
  Demux/6 -> Mux7/1
  Demux/7 -> Mux7/2
  Foot to COM Position [m m m]/1 -> select/1
  Foot to COM Velocity [m/s m/s m/s]/1 -> select1/1
  select/1 -> Mux21/1
  select1/1 -> Mux21/2
  Mux21/1 -> [Z_dZ_FootToCOM]
  Mux15/1 -> Z Flight Trajectory/1
  Mux5/1 -> Z Flight Trajectory/2
  [Z_dZ_FootToCOM] -> Mux6/4
  [Z_dZ_FootToCOM] -> Demux9/1
  Demux9/1 -> Mux15/1
  Demux9/2 -> Mux5/1
  Demux4/1 -> Mux15/2
  Demux4/2 -> Mux5/2
  Demux4/3 -> Terminator4/1
  Mux9/1 -> X Flight Trajectory/1
  Mux10/1 -> X Flight Trajectory/2
  Demux5/1 -> Mux9/1
  Demux5/2 -> Mux10/1
  Demux7/1 -> Mux9/2
  Demux7/2 -> Mux10/2
  [X_dX] -> Demux5/1
  Demux7/3 -> Terminator6/1
  Mux13/1 -> Y Flight Trajectory/1
  Mux12/1 -> Y Flight Trajectory/2
  Demux8/1 -> Mux13/1
  Demux8/2 -> Mux12/1
  Demux10/1 -> Mux13/2
  Demux10/2 -> Mux12/2
  [Y_dY] -> Demux8/1
  Demux10/3 -> Terminator7/1
  [CommandedX] -> Demux7/1
  [CommandedY] -> Demux10/1
  [CommandedZ] -> Demux4/1
  Generate Parabolic Foot Trajectories/3(Z_star) -> "Convert COM Position to Joint Angles + Leg Length "/4(Z_star), [CommandedZ]
  Mux3/1 -> Terminator/1

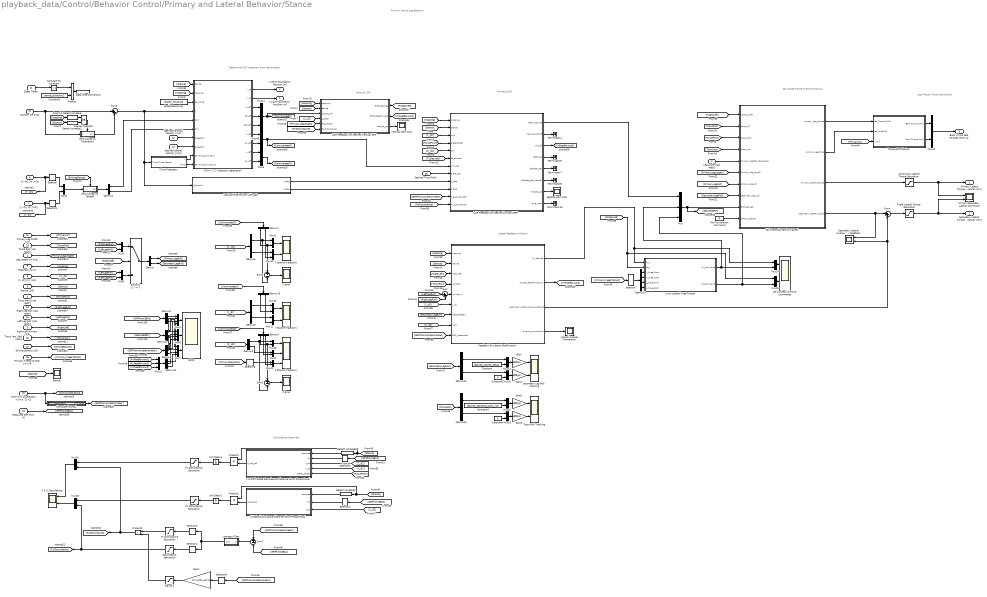
== system playback_data/Control/Behavior Control/Primary and Lateral Behavior/Stance ==
  note: Lateral feedback without Y
  note: 3D Yawed Frame Inverse Dynamics
  note: Forward LQR
  note: Vertical LQR
  note: Determine COM trajectory
      | from lookup table
  note: Primary Stance Leg Behavior
  note: Disturbance Observers
  note: Leg Torque / Force
      | Distribution
  Leg Length [m m/s] : Inport
  Torso Pitch [rad rad/s] : Inport  Port=2
  Stance [1/0] : Inport  Port=3
  Leg Angle [rad rad/s] : Inport  Port=4
  Right/Left Primary [1/0] : Inport  Port=5
  "[x, dx] [m, m/s]" : Inport  Port=6
  "[y, dy] [m, m/s]" : Inport  Port=7
  "[z, dz] [m, m/s]" : Inport  Port=8
  Hopping [1 or 0] : Inport  Port=9
  Measured GRF [N N N] : Inport  Port=10
  Steps Taken : Inport  Port=11
  Desired Forward Velocity [m/s] : Inport  Port=12
  Desired Lateral Velocity [m/s] : Inport  Port=13
  Right Leg Roll [rad rad/s] : Inport  Port=14
  Left Leg Roll [rad rad/s] : Inport  Port=15
  Torso Yaw [rad rad/s] : Inport  Port=16
  Exiting Stance [1/0] : Inport  Port=17
  Desired Torso Pitch : Inport  Port=18
  Torso Roll [rad rad/s] : Inport  Port=19
  COM XYZ Acceleration [m/s^2] x3 : Inport  Port=20
  System Time [s] : Inport  Port=21
  Primary Leg Width [m] : Inport  Port=22
  Primary Knees to Foot [m] x6 : Inport  Port=23
  3D Inverse Dynamics yawed : MATLAB Function  TreatAsAtomicUnit=on
  COM X,Y,Z  trajectory generation : MATLAB Function  TreatAsAtomicUnit=on
  Chirp Frequency : Subsystem
  Compare To Constant : simulink/Logic and Bit Operations/Compare To Constant  relop=<  const=1  OutDataTypeStr=uint8
  Compute Forces1 : Subsystem
  Constant : Constant  Value=desired_stance_beta2
  Constant1 : Constant  Value=0
  Constant2 : Constant  Value=stance_duration/2
  Constant3 : Constant  Value=desired_standing_torso_roll
  Constant4 : Constant  Value=0
  Continuous Lateral Torque Saturation : Saturate  UpperLimit=max_primary_lateral_stance_torque  LowerLimit=-max_primary_lateral_stance_torque
      settings: AttributesFormatString=Top: %<UpperLimit>\nBottom: %<LowerLimit>
  Data Type Conversion : DataTypeConversion  OutDataTypeStr=double
  Demux{,1,5,7..10,12..13} (9 alike) : Demux  Outputs=2
  Demux{2..4,6,11} (5 alike) : Demux  Outputs=3
  Demux14 : Demux
  Detect Increase{,1..3} (4 alike) : simulink/Logic and Bit Operations/Detect Increase  vinit=0.0  InputProcessing=Inherited  OutDataTypeStr=boolean
  "Disturbance Saturation " : Saturate  UpperLimit=100  LowerLimit=-100
      settings: AttributesFormatString=Top: %<UpperLimit>\nBottom: %<LowerLimit>
  Enable Bouncing : Constant  Value=enable_bouncing  SampleTime=sample_time
  Feedback for Lateral Stabilization : MATLAB Function  TreatAsAtomicUnit=on
  Flight Lateral Torque Saturation : Saturate  UpperLimit=HIP_MTR_MAX_CONT_TORQUE  LowerLimit=-HIP_MTR_MAX_CONT_TORQUE
      settings: AttributesFormatString=Top: %<UpperLimit>\nBottom: %<LowerLimit>
  Fx Disturbance Saturation : Saturate  UpperLimit=100  LowerLimit=-100
      settings: AttributesFormatString=Top: %<UpperLimit>\nBottom: %<LowerLimit>
  "Fx Disturbance Saturation " : Saturate  UpperLimit=100  LowerLimit=-100
      settings: AttributesFormatString=Top: %<UpperLimit>\nBottom: %<LowerLimit>
  Fz Disturbance Saturation : Saturate  UpperLimit=100  LowerLimit=-100
      settings: AttributesFormatString=Top: %<UpperLimit>\nBottom: %<LowerLimit>
  GRFs : Scope  NumInputPorts=3
      settings: TimeRange=12.737  YMin=-150~-200~0  YMax=200~150~1500  SampleInput=on
  Gain{,1..3} (4 alike) : Gain  Gain=180/pi
  Gain4 : Gain  Gain=2/(m_total_real*g)
  Hold Values on Takeoff : Subsystem
  Hold Values on Touchdown : Subsystem
  LQR Feedback for Desired Forward GRF : MATLAB Function  TreatAsAtomicUnit=on
  LQR Feedback for Desired Vertical GRF : MATLAB Function  TreatAsAtomicUnit=on
  Lateral Angular Momentum : Scope
      settings: YMin=-3.5  YMax=4  SaveName=ScopeData20  SampleInput=on
  Limit Lateral Knee Torque : MATLAB Function  TreatAsAtomicUnit=on
  Logical Operator : Logic  Operator=OR  AllPortsSameDT=off  OutDataTypeStr=boolean
  Lookup finite horizon LQR gain : MATLAB Function  TreatAsAtomicUnit=on
  Lowpass Filter : Subsystem  DialogController=fdesignblkfcn  InitFcn=fdesignblkfcn(gcbh, {'InitFcn'});  mask(Lowpass Filter){}
      mask help: Design a lowpass filter
      settings: CopyFcn=fdesignblkfcn(gcbh, {'CopyFcn'});
      mask Help: helpview(mapfilelocation('dsp'), 'dsplowpassfilter');
      mask Display: disp('Lowpass')
  Max of 1 : Saturate  UpperLimit=1  LowerLimit=0
      settings: AttributesFormatString=Top: %<UpperLimit>\nBottom: %<LowerLimit>
  Mux : Mux  Inputs=3
  Mux{1..3,5,8..10,12..20,22..25,49} (21 alike) : Mux  Inputs=2
  Mux11 : Mux  Inputs=3
  Mux21 : Mux  Inputs=3
  Mux4 : Mux
  Mux6 : Mux
  Mux7 : Mux
  Primary/Secondary Lateral Command : Scope  NumInputPorts=2
      settings: YMin=40~-5  YMax=150~5  SaveName=ScopeData25  SampleInput=on
  Product{,1..3} (4 alike) : Product
  QP Limited YZ Force Commands : Scope  NumInputPorts=2
      settings: YMin=40~-5  YMax=150~5  SaveName=ScopeData26  SampleInput=on
  Roll Accleration Command : Constant  Value=0
  Sagittal LQR Cost : Scope
      settings: YMin=22.5  YMax=62.5  SaveName=ScopeData10  SampleInput=on
  Secondary Lateral Inverse Dynamics / Feedback : Scope  NumInputPorts=2
      settings: YMin=-3.5~-5  YMax=4~5  SaveName=ScopeData9  SampleInput=on
  Secondary Leg Roll Tracking : Scope  NumInputPorts=2
      settings: YMin=-3.5~-5  YMax=4~5  SaveName=ScopeData12  SampleInput=on
  Selector : Selector  InputPortWidth=2  Indices=[2]
  Selector1 : Selector  InputPortWidth=2  Indices=[2]
  Selector{2,4,6,8} (4 alike) : Selector  InputPortWidth=3  Indices=[3]
  Selector3 : Selector  InputPortWidth=3  Indices=[1]
  Selector5 : Selector  InputPortWidth=3  Indices=[1]
  Selector7 : Selector  InputPortWidth=6  Indices=[2 5 3 6]
  Stance : Scope
      settings: YMin=-0.05  YMax=0.11  SaveName=stance_time_history  SampleInput=on
  Sum : Sum  Inputs=|+-
  Sum2 : Sum  Inputs=|+-
  Sum4 : Sum  Inputs=|++
  Sum5 : Sum  Inputs=+-
  Sum6 : Sum  Inputs=+-
  Sum7 : Sum  Inputs=+-
  Switch1 : Switch  Criteria=u2 ~= 0
  Terminator{4,6..8,10} (5 alike) : Terminator
  Torque Distribution : Subsystem
  Torso Roll Tracking : Scope  NumInputPorts=2
      settings: YMin=-3.5~-5  YMax=4~5  SaveName=ScopeData15  SampleInput=on
  Unit Delay1 : UnitDelay  SampleTime=sample_time
  Unit Delay2 : UnitDelay  SampleTime=sample_time
  Vertical LQR Cost : Scope
      settings: YMin=11  YMax=16  SaveName=ScopeData18  SampleInput=on
  X & Pitch State Disturbance Observer Error-Proportional : MATLAB Function  TreatAsAtomicUnit=on
  X & Z Disturbance : Scope  NumInputPorts=2
      settings: YMin=-125~-800  YMax=175~700  SaveName=ScopeData16  SampleInput=on
  X Stance Trajectory : Scope  NumInputPorts=2
      settings: YMin=0~-0.02  YMax=0.005~0.03  SaveName=ScopeData8  SampleInput=on
  X error : Scope
      settings: YMin=-0.05  YMax=0.11  SaveName=ScopeData24  SampleInput=on
  Y Stance Trajectory : Scope  NumInputPorts=2
      settings: YMin=0.005~-0.5  YMax=0.1~0.3  SaveName=ScopeData5  SampleInput=on
  Z Error : Scope
      settings: YMin=-0.007  YMax=0.0005  SaveName=ScopeData23  SampleInput=on
  Z Stance Trajectory : Scope  NumInputPorts=3
      settings: YMin=0.85~-0.4~-3  YMax=0.98~0.6~11  SaveName=z_stance_trajectory  SampleInput=on
  Z State Disturbance Observer Error-Proportional : MATLAB Function  TreatAsAtomicUnit=on
  Primary Lateral Torque Command (stance) [Nm] : Outport
  Secondary Lateral Torque Command (stance) [Nm] : Outport  Port=2
  Back / Front SEA Torques [Nm] x2 : Outport  Port=3
  X COM Touchdown Position [m] : Outport  Port=4
  Y COM Touchdown Position [m] : Outport  Port=5
  wires:
  Fz Disturbance Saturation/1 -> Mux19/1
  Selector5/1 -> "Fx Disturbance Saturation "/1
  "Disturbance Saturation "/1 -> [FzDisturbance], Mux19/2
  Max of 1/1 -> Product3/2
  "Fx Disturbance Saturation "/1 -> Product3/1
  Gain4/1 -> Max of 1/1
  Selector8/1 -> Gain4/1
  [GRFfromAccelerometer] -> Selector8/1
  Limit Lateral Knee Torque/2(Fz_command) -> Mux/3, Mux25/2
  [FzDisturbance] -> LQR Feedback for Desired Vertical GRF/6(Fz_disturbance)
  [FxDisturbance] -> LQR Feedback for Desired Forward GRF/12(Fx_disturbance)
  Lowpass Filter/1(Out) -> Selector5/1, Selector4/1
  Chirp Frequency/2(dw/dt) -> COM X,Y,Z  trajectory generation/10(standing_bounce_dw)
  [Stance] -> Stance/1
  Chirp Frequency/1(w) -> COM X,Y,Z  trajectory generation/9(standing_bounce_w)
  Selector2/1 -> Z State Disturbance Observer Error-Proportional/2(Fz)
  Sum7/1 -> Lowpass Filter/1(In)
  Product3/1 -> Mux20/2, [FxDisturbance]
  Mux20/1 -> X & Z Disturbance/1
  [GRFfromAccelerometer] -> Sum7/1
  Sum6/1 -> X error/1
  Demux7/1 -> Mux9/2, Sum6/1
  Demux5/1 -> Mux9/1, Sum6/2
  Unit Delay2/1 -> Fz Disturbance Saturation/1
  Unit Delay1/1 -> Fx Disturbance Saturation/1
  Selector3/1 -> X & Pitch State Disturbance Observer Error-Proportional/2(Fx)
  Fx Disturbance Saturation/1 -> Mux20/1
  Enable Bouncing/1 -> COM X,Y,Z  trajectory generation/3(bouncing)
  [RightLeft] -> Feedback for Lateral Stabilization/3(right_left)
  Constant4/1 -> Mux18/2
  Mux18/1 -> Gain3/1
  Demux13/2 -> Mux18/1
  Constant3/1 -> Mux17/2
  Demux13/1 -> Mux17/1
  Mux17/1 -> Gain2/1
  Gain3/1 -> Torso Roll Tracking/2
  Gain2/1 -> Torso Roll Tracking/1
  [TorsoRoll] -> Demux13/1
  Constant1/1 -> Mux16/2
  Demux12/2 -> Mux16/1
  Mux16/1 -> Gain1/1
  Gain1/1 -> Secondary Leg Roll Tracking/2
  Gain/1 -> Secondary Leg Roll Tracking/1
  Constant/1 -> Mux14/2
  Demux12/1 -> Mux14/1
  Mux14/1 -> Gain/1
  [SecondaryLegRoll] -> Demux12/1
  Feedback for Lateral Stabilization/3(secondary_lateral_torque_desired) -> Sum4/2, Secondary Lateral Inverse Dynamics / Feedback/2
  Sum4/1 -> Flight Lateral Torque Saturation/1
  3D Inverse Dynamics yawed/3(primary_lateral_torque) -> Continuous Lateral Torque Saturation/1
  3D Inverse Dynamics yawed/4(secondary_lateral_torque) -> Secondary Lateral Inverse Dynamics / Feedback/1, Sum4/1
  Sum/1 -> Feedback for Lateral Stabilization/5(symdsym)
  [SecondaryLegRoll] -> Feedback for Lateral Stabilization/7(beta2dbeta2)
  [Y_dY] -> Feedback for Lateral Stabilization/6(y_dy)
  [RightLegRoll] -> Sum/2
  [LeftLegRoll] -> Sum/1
  Roll Accleration Command/1 -> 3D Inverse Dynamics yawed/10(ddRoll_desired)
  Feedback for Lateral Stabilization/1(Fy_desired) -> Limit Lateral Knee Torque/1(Fy_s), Mux24/1
  Continuous Lateral Torque Saturation/1 -> Primary/Secondary Lateral Command/1, Primary Lateral Torque Command (stance) [Nm]/1
  Demux11/3 -> Mux7/4
  Demux11/2 -> Mux6/4
  Demux11/1 -> Mux4/4
  Mux/1 -> [DesiredGRF], 3D Inverse Dynamics yawed/9(GRF_desired)
  LQR Feedback for Desired Forward GRF/1(GRFx_desired) -> Mux/1
  Left Leg Roll [rad rad/s]/1 -> [LeftLegRoll]
  Right/Left Primary [1/0]/1 -> [RightLeft]
  [CommandedY] -> Demux10/1
  [CommandedX] -> Demux7/1
  [Y_dY] -> Demux8/1
  Demux10/2 -> Mux12/2
  Demux10/1 -> Mux13/2
  Demux8/2 -> Mux12/1
  Demux8/1 -> Mux13/1
  Mux12/1 -> Y Stance Trajectory/2
  Mux13/1 -> Y Stance Trajectory/1
  [X_dX] -> Demux5/1
  Demux7/2 -> Mux10/2
  Demux5/2 -> Mux10/1
  Mux10/1 -> X Stance Trajectory/2
  Mux9/1 -> X Stance Trajectory/1
  Demux3/3 -> Mux7/2
  Demux3/2 -> Mux6/2
  Demux3/1 -> Mux4/2
  Demux2/3 -> Mux7/1
  Demux2/2 -> Mux6/1
  Mux7/1 -> GRFs/3
  Mux6/1 -> GRFs/2
  Demux2/1 -> Mux4/1
  Mux4/1 -> GRFs/1
  [DesiredGRF] -> Demux3/1
  [GRFfromSEAs] -> Demux2/1
  Torso Roll [rad rad/s]/1 -> [TorsoRoll]
  [PrimaryLegLength] -> LQR Feedback for Desired Vertical GRF/5(leg_length)
  Leg Length [m m/s]/1 -> [PrimaryLegLength]
  System Time [s]/1 -> Sum2/1, Hold Values on Touchdown/1(in)
  [GRFfromAccelerometer] -> Feedback for Lateral Stabilization/9(GRF_measured)
  [Hopping] -> Feedback for Lateral Stabilization/1(hopping)
  [ExitingStance] -> Hold Values on Takeoff/Trigger
  Exiting Stance [1/0]/1 -> [ExitingStance]
  Torso Yaw [rad rad/s]/1 -> [TorsoYaw]
  Desired Lateral Velocity [m/s]/1 -> COM X,Y,Z  trajectory generation/8(target_DY)
  Selector1/1 -> Mux3/2
  Hold Values on Takeoff/1(out) -> Demux1/1
  Mux3/1 -> Hold Values on Takeoff/1(in)
  "[y, dy] [m, m/s]"/1 -> Selector1/1, [Y_dY]
  [RightLeft] -> Switch1/2
  [RightLegRoll] -> Mux2/2
  [LeftLegRoll] -> Mux2/1
  [LeftLegRoll] -> Mux1/2
  [RightLegRoll] -> Mux1/1
  Right Leg Roll [rad rad/s]/1 -> [RightLegRoll]
  Mux2/1 -> Switch1/3
  Mux1/1 -> Switch1/1
  Demux/1 -> [PrimaryLegRoll]
  Demux/2 -> [SecondaryLegRoll]
  Switch1/1 -> Demux/1
  [PrimaryLegRoll] -> 3D Inverse Dynamics yawed/7(primary_leg_roll)
  [SecondaryLegRoll] -> 3D Inverse Dynamics yawed/8(secondary_leg_roll)
  Leg Angle [rad rad/s]/1 -> 3D Inverse Dynamics yawed/5(primary_sagittal_leg_angle)
  [PrimaryLegLength] -> 3D Inverse Dynamics yawed/6(primary_leg_length)
  [TorsoYaw] -> 3D Inverse Dynamics yawed/4(torso_yaw)
  [TorsoRoll] -> 3D Inverse Dynamics yawed/2(torso_roll)
  [TorsoPitch] -> 3D Inverse Dynamics yawed/3(torso_pitch)
  Mux5/1 -> [CommandedY]
  COM X,Y,Z  trajectory generation/2(y_0) -> Y COM Touchdown Position [m]/1
  [TorsoRoll] -> Feedback for Lateral Stabilization/4(rolldroll)
  [Stance] -> Feedback for Lateral Stabilization/2(stance)
  [Hopping] -> LQR Feedback for Desired Vertical GRF/1(hopping)
  Selector/1 -> Mux3/1
  Demux1/1 -> COM X,Y,Z  trajectory generation/5(dx0)
  [Stance] -> Detect Increase1/1
  [Hopping] -> Detect Increase/1
  Compare To Constant/1 -> Product/1
  Detect Increase1/1 -> Logical Operator/2
  Detect Increase/1 -> Logical Operator/1
  Constant2/1 -> Product/2
  Product/1 -> Data Type Conversion/1
  Steps Taken/1 -> Compare To Constant/1
  [GRFfromAccelerometer] -> LQR Feedback for Desired Forward GRF/11(measured_GRF)
  Measured GRF [N N N]/1 -> [GRFfromSEAs]
  [Hopping] -> LQR Feedback for Desired Forward GRF/1(hopping)
  [Hopping] -> COM X,Y,Z  trajectory generation/2(hopping)
  Hopping [1 or 0]/1 -> [Hopping]
  [RightLeft] -> 3D Inverse Dynamics yawed/1(right_or_left)
  Torso Pitch [rad rad/s]/1 -> [TorsoPitch]
  LQR Feedback for Desired Forward GRF/8(ang_mom) -> Terminator10/1
  LQR Feedback for Desired Forward GRF/7(cost_to_go) -> Sagittal LQR Cost/1
  LQR Feedback for Desired Forward GRF/6(ddtheta_star_neutral) -> Terminator8/1
  LQR Feedback for Desired Forward GRF/5(ddtheta_star) -> Terminator7/1
  LQR Feedback for Desired Vertical GRF/3(cost_to_go) -> Vertical LQR Cost/1
  Demux1/2 -> COM X,Y,Z  trajectory generation/6(dy0)
  "[x, dx] [m, m/s]"/1 -> Selector/1, [X_dX]
  Logical Operator/1 -> Hold Values on Touchdown/Trigger
  [Stance] -> LQR Feedback for Desired Vertical GRF/2(stance)
  Stance [1/0]/1 -> [Stance]
  Hold Values on Touchdown/1(out) -> Sum2/2
  LQR Feedback for Desired Vertical GRF/1(GRFz_desired) -> [FzDesired]
  Sum2/1 -> Chirp Frequency/1(Time Since Stance), Lookup finite horizon LQR gain/1(t_forward), COM X,Y,Z  trajectory generation/4(t)
  Desired Forward Velocity [m/s]/1 -> COM X,Y,Z  trajectory generation/7(target_DX)
  [Z_dZ] -> LQR Feedback for Desired Forward GRF/5(zdz)
  Lookup finite horizon LQR gain/1(K_sag) -> LQR Feedback for Desired Forward GRF/9(K_sag)
  Desired Torso Pitch/1 -> LQR Feedback for Desired Forward GRF/8(theta_star)
  Mux49/1 -> LQR Feedback for Desired Forward GRF/7(xdx_ref), [CommandedX]
  [TorsoPitch] -> LQR Feedback for Desired Forward GRF/4(thetadtheta)
  [X_dX] -> LQR Feedback for Desired Forward GRF/3(xdx)
  Mux11/1 -> LQR Feedback for Desired Vertical GRF/3(zdzddz_ref), [CommandedZ]
  COM X,Y,Z  trajectory generation/5(ddz_ref) -> Mux11/3
  COM X,Y,Z  trajectory generation/4(dz_ref) -> Mux11/2
  COM X,Y,Z  trajectory generation/1(x_0) -> X COM Touchdown Position [m]/1
  COM X,Y,Z  trajectory generation/9(dy_ref) -> Mux5/2
  COM X,Y,Z  trajectory generation/8(y_ref) -> Mux5/1
  COM X,Y,Z  trajectory generation/7(dx_ref) -> Mux49/2
  COM X,Y,Z  trajectory generation/6(x_ref) -> Mux49/1
  [Stance] -> LQR Feedback for Desired Forward GRF/2(stance)
  COM X,Y,Z  trajectory generation/3(z_ref) -> Mux11/1
  [Z_dZ] -> LQR Feedback for Desired Vertical GRF/4(z_state)
  Lookup finite horizon LQR gain/2(P_sag) -> LQR Feedback for Desired Forward GRF/10(P_sag)
  [Stance] -> COM X,Y,Z  trajectory generation/1(stance)
  LQR Feedback for Desired Forward GRF/4(GRFx_lqr) -> Terminator6/1
  Feedback for Lateral Stabilization/4(angular_momentum) -> Lateral Angular Momentum/1
  Demux6/1 -> Mux4/3
  Demux6/2 -> Mux6/3
  Demux6/3 -> Mux7/3
  Flight Lateral Torque Saturation/1 -> Primary/Secondary Lateral Command/2, Secondary Lateral Torque Command (stance) [Nm]/1
  "[z, dz] [m, m/s]"/1 -> [Z_dZ]
  [Z_dZ] -> X & Pitch State Disturbance Observer Error-Proportional/3(z_dz)
  [TorsoPitch] -> X & Pitch State Disturbance Observer Error-Proportional/5(theta_dtheta)
  [X_dX] -> X & Pitch State Disturbance Observer Error-Proportional/4(x_dx)
  [GRFfromSEAs] -> Selector3/1
  Detect Increase3/1 -> X & Pitch State Disturbance Observer Error-Proportional/1(enabled)
  Detect Increase2/1 -> Z State Disturbance Observer Error-Proportional/1(enabled)
  [GRFfromSEAs] -> Selector2/1
  [Z_dZ] -> Z State Disturbance Observer Error-Proportional/3(z_dz)
  Product1/1 -> Unit Delay1/1
  Product2/1 -> Unit Delay2/1
  X & Pitch State Disturbance Observer Error-Proportional/1(d_hat_tp1) -> Product1/2
  [Stance] -> Product1/1, Detect Increase3/1
  Z State Disturbance Observer Error-Proportional/1(d_hat_tp1) -> Product2/2
  [Stance] -> Product2/1, Detect Increase2/1
  Mux19/1 -> X & Z Disturbance/2
  [GRFfromSEAs] -> Sum7/2
  Selector4/1 -> "Disturbance Saturation "/1
  COM XYZ Acceleration [m/s^2] x3/1 -> Compute Forces1/1(XYZ Acceleration), [ComAcceleration]
  [GRFfromAccelerometer] -> Demux6/1
  LQR Feedback for Desired Vertical GRF/2(GRFz_feedforward) -> [FzFeedforward]
  Mux21/1 -> Demux11/1
  [FzFeedforward] -> Mux21/3
  Mux15/1 -> Z Stance Trajectory/1
  Mux8/1 -> Z Stance Trajectory/2
  [Z_dZ] -> Demux9/1
  Demux9/1 -> Mux15/1, Sum5/2
  Demux9/2 -> Mux8/1
  Demux4/1 -> Mux15/2, Sum5/1
  Demux4/2 -> Mux8/2
  Demux4/3 -> Mux22/2
  [CommandedZ] -> Demux4/1
  Sum5/1 -> Z Error/1
  Mux22/1 -> Z Stance Trajectory/3
  [ComAcceleration] -> Selector6/1
  Selector6/1 -> Mux22/1
  3D Inverse Dynamics yawed/1(primary_leg_torque) -> Torque Distribution/1(Leg Torque [Nm])
  [PrimaryW] -> Torque Distribution/3(w [m])
  3D Inverse Dynamics yawed/2(primary_leg_force) -> Torque Distribution/2(Leg Force [N])
  Primary Leg Width [m]/1 -> [PrimaryW]
  Torque Distribution/1(Back Torque [Nm]) -> Mux23/1
  Torque Distribution/2(Front Torque [Nm]) -> Mux23/2
  Mux23/1 -> Back / Front SEA Torques [Nm] x2/1
  [FxFeedforward] -> Mux21/1
  [FzDesired] -> LQR Feedback for Desired Forward GRF/6(Fz_desired)
  [FzDesired] -> Limit Lateral Knee Torque/2(Fz_s), Mux25/1
  [Z_dZ] -> Feedback for Lateral Stabilization/8(z_dz)
  [FyFeedforward] -> Mux21/2
  Compute Forces1/1(XYZ Force) -> [GRFfromAccelerometer]
  LQR Feedback for Desired Forward GRF/3(true_ff) -> [FxFeedforward]
  LQR Feedback for Desired Forward GRF/2(netural_pitch_ff) -> Terminator4/1
  Feedback for Lateral Stabilization/2(neutral_feedforward_Fy) -> [FyFeedforward]
  Primary Knees to Foot [m] x6/1 -> [PrimaryKneesToFoot]
  [PrimaryKneesToFoot] -> Selector7/1
  Demux14/1 -> Limit Lateral Knee Torque/3(y_knee_front)
  Demux14/2 -> Limit Lateral Knee Torque/4(y_knee_back)
  Demux14/3 -> Limit Lateral Knee Torque/5(z_knee_front)
  Demux14/4 -> Limit Lateral Knee Torque/6(z_knee_back)
  Selector7/1 -> Demux14/1
  Mux24/1 -> QP Limited YZ Force Commands/1
  Mux25/1 -> QP Limited YZ Force Commands/2
  Limit Lateral Knee Torque/1(Fy_command) -> Mux24/2, Mux/2
